simulink model "funtransfer"  (Simulink 7.5)
settings: Solver=ode4  StartTime=0.0  StopTime=3  FixedStep=1.2207e-004  RelTol=1e-3
settings Model: Creator=Leonardo  LastModifiedBy=Leo
settings OptimizationCC: InlineInvariantSignals=on  InitFltsAndDblsToZero=on
settings DebuggingCC: SaveWithParameterizedLinksMsg=none  SignalResolutionControl=TryResolveAllWithWarning  MultiTaskDSMMsg=warning  MultiTaskCondExecSysMsg=none  StrictBusMsg=None
settings RTWCC: IncludeERTFirstTime=on
settings GRTTargetCC: TargetFcnLib=ansi_tfl_tmw.mat

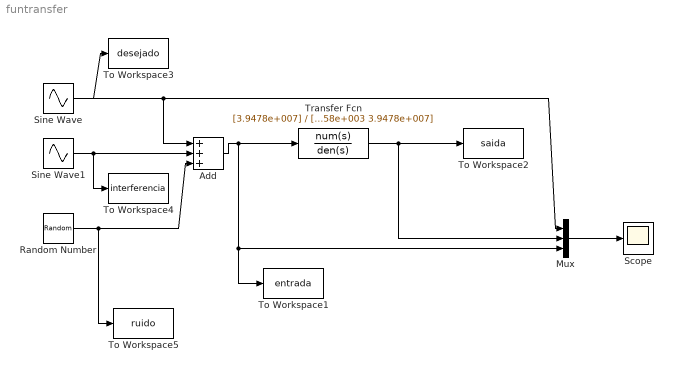
== system funtransfer ==
  Add : Sum  Inputs=+++  OutDataType=fixdt(1, 16)  OutScaling=2^-10
  Mux : Mux  Inputs=3
  Random Number : RandomNumber  Variance=0.01  SampleTime=0
  Scope : Scope
      settings: MaxDataPoints=50000
  Sine Wave : Sin  Amplitude=sqrt(2)  Bias=0  Frequency=3.1416e+003  Phase=0  Samples=10  SampleTime=0  Offset=0
  Sine Wave1 : Sin  Amplitude=sqrt(2)  Bias=0  Frequency=3.1416e+004  Phase=0  Samples=10  SampleTime=0  Offset=0
  To Workspace1 : ToWorkspace  VariableName=entrada  SaveFormat=Structure With Time
  To Workspace2 : ToWorkspace  VariableName=saida  SaveFormat=Structure With Time
  To Workspace3 : ToWorkspace  VariableName=desejado  SaveFormat=Structure With Time
  To Workspace4 : ToWorkspace  VariableName=interferencia  SaveFormat=Structure With Time
  To Workspace5 : ToWorkspace  VariableName=ruido  SaveFormat=Structure With Time
  Transfer Fcn : TransferFcn  Numerator=[3.9478e+007]  Denominator=[1 8.8858e+003 3.9478e+007]
  wires:
  Mux/1 -> Scope/1
  Transfer Fcn/1 -> To Workspace2/1, Mux/2
  Add/1 -> Mux/3, To Workspace1/1, Transfer Fcn/1
  Sine Wave/1 -> Add/1, Mux/1, To Workspace3/1
  Random Number/1 -> Add/3, To Workspace5/1
  Sine Wave1/1 -> Add/2, To Workspace4/1
